simulink model "Exp3_1_SimModel"  (R2014b)
settings: Solver=ode45  StartTime=1  StopTime=1.5  RelTol=1e-3
values from neighbouring files (symbols this model uses):
  i_ref = 1000    [Exp3_1_SimCode.m]
  ki = 1.176    [Exp3_1_SimCode.m]
  kp = 0.138    [Exp3_1_SimCode.m]
  R = 5e-3    (= 0.005)    [Exp2_1.m]    (also in Exp2_1_SimCode.m; Exp3_1_SimCode.m = 0.00588)
  Ts = 1e-5    (= 1e-05)    [Exp2_1_SimCode.m]    (also in Exp3_1_SimCode.m)
  V_DC = 605 * 2    (= 1210)    [Exp2_1.m]    (also in Exp2_1_SimCode.m; Exp3_1_SimCode.m = 1200)
  V_s = 415    [Exp2_1.m]    (also in Exp2_1_SimCode.m = 400; Exp3_1_SimCode.m = 400)
libraries: powerlib x12, simulink x1, powerlib_meascontrol x1
settings Model: Creator=tommy  LastModifiedBy=tommy
settings DataIOCC: FinalStateName=xFinal_1  InitialState=xFinal_0  LoadInitialState=on  SaveFinalState=on  SaveCompleteFinalSimState=on

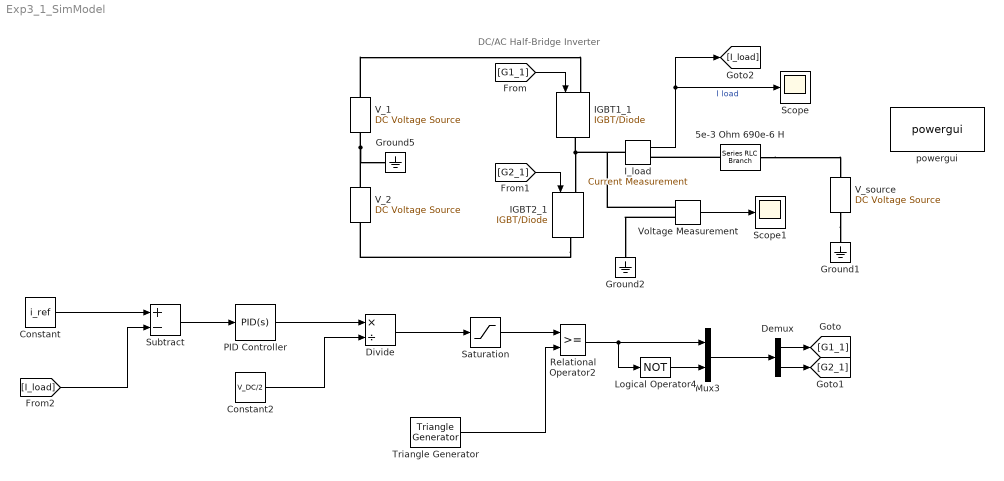
== system Exp3_1_SimModel ==
  note: DC/AC Half-Bridge Inverter
  5e-3 Ohm 690e-6 H : powerlib/Elements/Series RLC Branch  LConnTagsString=__new0  RConnTagsString=__new0  BranchType=RL  Resistance=R  Inductance=690e-6  SetiL0=off  InitialCurrent=1.6e3  Capacitance=[]  Setx0=off  InitialVoltage=0  Measurements=None
  Constant : Constant  Value=i_ref
  Constant2 : Constant  Value=V_DC/2
  Demux : Demux  Outputs=2
  Divide : Product  Inputs=*/
  Ground1 : powerlib/Elements/Ground  LConnTagsString=a
  Ground2 : powerlib/Elements/Ground  LConnTagsString=a
  Ground5 : powerlib/Elements/Ground  LConnTagsString=a
  IGBT1_1 : powerlib/Power Electronics/IGBT//Diode  Ron=1e-6  Rs=1e5  Cs=inf  Measurements=off
  IGBT2_1 : powerlib/Power Electronics/IGBT//Diode  Ron=1e-6  Rs=1e5  Cs=inf  Measurements=off
  I_load : powerlib/Measurements/Current Measurement  Tag=PoWeRsYsTeMmEaSuReMeNt  PhasorSimulation=off  OutputType=Magnitude  PSBequivalent=0
  Logical Operator4 : Logic  Operator=NOT
  Mux3 : Mux  Inputs=2
  PID Controller : simulink/Continuous/PID Controller  Controller=PID  TimeDomain=Continuous-time  SampleTime=-1  IntegratorMethod=Forward Euler  FilterMethod=Forward Euler  Form=Parallel  P=kp  I=ki  D=0  N=0  InitialConditionSource=internal  InitialConditionForIntegrator=0  InitialConditionForFilter=0  ExternalReset=none  LimitOutput=off  UpperSaturationLimit=inf  LowerSaturationLimit=-inf  LinearizeAsGain=on  AntiWindupMode=none  Kb=1  TrackingMode=off  Kt=1  PParamMin=[]  PParamMax=[]  IParamMin=[]  IParamMax=[]  DParamMin=[]  DParamMax=[]  NParamMin=[]  NParamMax=[]  KbParamMin=[]  KbParamMax=[]  KtParamMin=[]  KtParamMax=[]  POutMin=[]  POutMax=[]  IOutMin=[]  IOutMax=[]  DOutMin=[]  DOutMax=[]  NOutMin=[]  NOutMax=[]  KbOutMin=[]  KbOutMax=[]  KtOutMin=[]  KtOutMax=[]  IntegratorOutMin=[]  IntegratorOutMax=[]  FilterOutMin=[]  FilterOutMax=[]  SumOutMin=[]  SumOutMax=[]  SumI1OutMin=[]  SumI1OutMax=[]  SumI2OutMin=[]  SumI2OutMax=[]  SumI3OutMin=[]  SumI3OutMax=[]  SumDOutMin=[]  SumDOutMax=[]  SaturationOutMin=[]  SaturationOutMax=[]  IntegratorContinuousStateAttributes=''  IntegratorStateMustResolveToSignalObject=off  IntegratorRTWStateStorageClass=Auto  FilterContinuousStateAttributes=''  FilterStateMustResolveToSignalObject=off  FilterRTWStateStorageClass=Auto  DifferentiatorICPrevScaledInput=0  DifferentiatorOutMin=[]  DifferentiatorOutMax=[]  UseFilter=on
  Relational Operator2 : RelationalOperator  OutDataTypeStr=boolean  ZeroCross=off  InputSameDT=on
  Saturation : Saturate  UpperLimit=1  LowerLimit=-1
  Scope : Scope
      settings: TimeRange=0.1489795918367347  YMin=3534.36018957346  YMax=4174.170616113744  SaveName=I_load
  Scope1 : Scope
      settings: YMin=0  YMax=35000
  Subtract : Sum  Inputs=+-
  Triangle Generator : powerlib_meascontrol/Pulse & Signal Generators/Triangle Generator  Freq=54*60  Phase=0  Ts=0
  V_1 : powerlib/Electrical Sources/DC Voltage Source  Description=source block  Amplitude=V_DC/2  Measurements=None
      settings: AttributesFormatString=\n
  V_2 : powerlib/Electrical Sources/DC Voltage Source  Description=source block  Amplitude=V_DC/2  Measurements=None
      settings: AttributesFormatString=\n
  V_source : powerlib/Electrical Sources/DC Voltage Source  Amplitude=V_s  Measurements=None
  Voltage Measurement : powerlib/Measurements/Voltage Measurement  PhasorSimulation=off  OutputType=Complex  PSBequivalent=0
  powergui : powerlib/powergui  SimulationMode=Discrete  SolverType=Tustin/Backward Euler (TBE)  SampleTime=Ts  frequency=60  SPID=off  DisableSnubberDevices=off  DisableRonSwitches=off  DisableVfSwitches=off  SwTol=0  DisplayEquations=off  Interpol=off  methode=off  Ts=0  frequencyindice=0  Pbase=100e6  ErrMax=1e-4  Iterations=50  UnitsV=kV  UnitsW=MW  FunctionMessages=off  echomessages=off  HookPort=off  EnableUseOfTLC=off  x0status=blocks  RestoreLinks=warning  ResistiveCurrentMeasurement=off  Frange=[0:2:500]  Ylog=off  Xlog=on  ShowGrid=off  save=off  variable=ZData  structure=sps1phPWM1_str  ZoomFFT=on  StartTime=0.1-2/60  cycles=2  DisplayStyle=1  fundamental=60  FreqAxis=off  MaxFrequency=5000  frequencyindicesteady=1  RmsSteady=1  display=off
  wires:
  [G1_1] -> IGBT1_1/1
  [G2_1] -> IGBT2_1/1
  Demux/1 -> [G1_1]
  Demux/2 -> [G2_1]
  I_load/1 -> [I_load], Scope/1  "I load"
  Voltage Measurement/1 -> Scope1/1
  Triangle Generator/1 -> Relational Operator2/2
  Logical Operator4/1 -> Mux3/2
  Mux3/1 -> Demux/1
  Relational Operator2/1 -> Logical Operator4/1, Mux3/1
  Constant/1 -> Subtract/1
  [I_load] -> Subtract/2
  Subtract/1 -> PID Controller/1
  PID Controller/1 -> Divide/1
  Divide/1 -> Saturation/1
  Saturation/1 -> Relational Operator2/1
  Constant2/1 -> Divide/2
  connections:
  V_1/LConn1 -- V_2/RConn1 -- Ground5/LConn1
  IGBT1_1/RConn1 -- Voltage Measurement/LConn1 -- I_load/LConn1 -- IGBT2_1/LConn1
  IGBT2_1/RConn1 -- V_2/LConn1
  V_1/RConn1 -- IGBT1_1/LConn1
  5e-3 Ohm 690e-6 H/RConn1 -- I_load/RConn1
  V_source/LConn1 -- Ground1/LConn1
  5e-3 Ohm 690e-6 H/LConn1 -- V_source/RConn1
  Voltage Measurement/LConn2 -- Ground2/LConn1
